simulink model "model"  (R2022b)
settings: Solver=VariableStepAuto  StartTime=0.0  StopTime=10.0  RelTol=1e-3
settings Model: Creator=markm  LastModifiedBy=markm

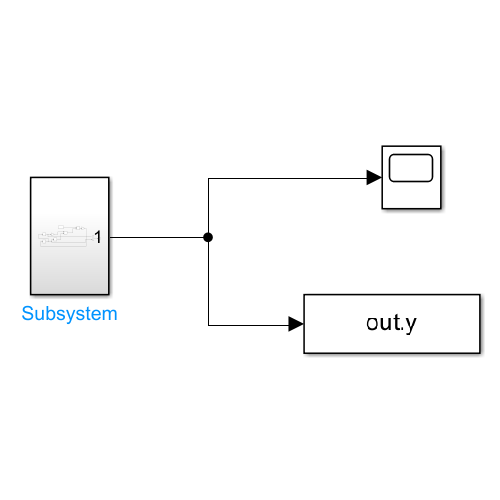
[thumbnail: Simulink's stored preview of the top-level diagram]
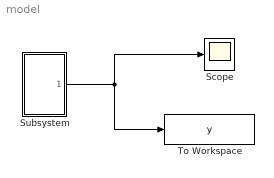
== system model ==
  Scope : Scope
  Subsystem : Subsystem
  To Workspace : ToWorkspace  VariableName=y  SaveFormat=Timeseries  SampleTime=-1
  wires:
  Subsystem/1(Solving) -> To Workspace/1, Scope/1

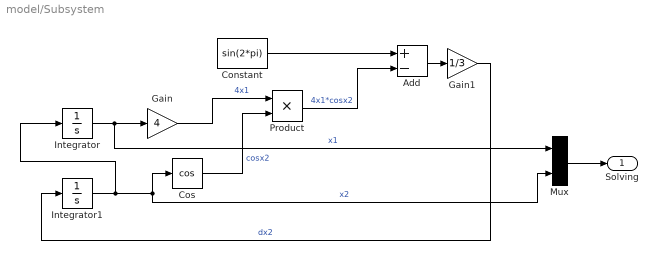
== system model/Subsystem ==
  Add : Sum  Inputs=+-
  Constant : Constant  Value=sin(2*pi)
  Cos : Trigonometry  Operator=cos
  Gain : Gain  Gain=4
  Gain1 : Gain  Gain=1/3
  Integrator : Integrator  InitialCondition=1
  Integrator1 : Integrator
  Mux : Mux  Inputs=2
  Product : Product
  Solving : Outport
  wires:
  Constant/1 -> Add/1
  Gain/1 -> Product/1  "4x1"
  Integrator1/1 -> Mux/2, Cos/1, Integrator/1  "x2"
  Cos/1 -> Product/2  "cosx2"
  Add/1 -> Gain1/1
  Product/1 -> Add/2  "4x1*cosx2"
  Integrator/1 -> Mux/1, Gain/1  "x1"
  Gain1/1 -> Integrator1/1  "dx2"
  Mux/1 -> Solving/1
